simulink model "PID_controller_lat_stage1_plot"  (R2019a)
settings: Solver=VariableStepAuto  StartTime=0.0  StopTime=100  FixedStep=1e-4  RelTol=1e-5
undefined symbols (not defined in the file): sys
libraries: aerolibactuator x1, simulink x1
settings Model: Creator=tyson  LastModifiedBy=tyson
settings DebuggingCC: TimeAdjustmentMsg=warning

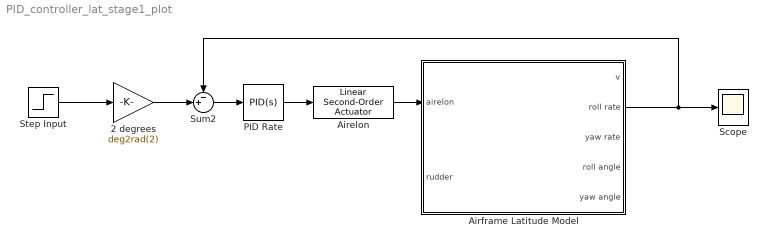
== system PID_controller_lat_stage1_plot ==
  2 degrees : Gain  Gain=deg2rad(2)
  Airelon : aerolibactuator/Linear Second-Order Actuator  wn_fin=actuators.naturalFreq  z_fin=actuators.dampingRatio  fin_act_0=0  fin_act_vel=0
      settings: SourceProductName=Aerospace Blockset  SourceProductBaseCode=AE
  Airframe Latitude Model : Subsystem
      mask Display: image('/home/tyson/Dropbox/Academic/4th Year/ELEN4011/matlab/icons/airframe_lat.png');
  PID Rate : simulink/Continuous/PID Controller  Controller=PID  Form=Parallel  TimeDomain=Continuous-time  SampleTime=-1  IntegratorMethod=Forward Euler  FilterMethod=Forward Euler  ControllerParametersSource=internal  P=0.088381890868231  I=0.0632480324268729  D=-0.40850773748129  UseFilter=on  N=0.167390609816389  TunerSelectOption=Transfer Function Based (PID Tuner App)  InitialConditionSource=internal  InitialConditionForIntegrator=0  InitialConditionForFilter=0  DifferentiatorICPrevScaledInput=0  ExternalReset=none  TrackingMode=off  Kt=1  LimitOutput=off  UpperSaturationLimit=pi  LowerSaturationLimit=-pi  LinearizeAsGain=on  AntiWindupMode=clamping  Kb=1  POutMin=[]  POutMax=[]  IOutMin=[]  IOutMax=[]  DOutMin=[]  DOutMax=[]  NOutMin=[]  NOutMax=[]  SumOutMin=[]  SumOutMax=[]  SaturationOutMin=[]  SaturationOutMax=[]  PParamMin=[]  PParamMax=[]  IParamMin=[]  IParamMax=[]  DParamMin=[]  DParamMax=[]  NParamMin=[]  NParamMax=[]  KbParamMin=[]  KbParamMax=[]  KtParamMin=[]  KtParamMax=[]  KbOutMin=[]  KbOutMax=[]  KtOutMin=[]  KtOutMax=[]  IntegratorOutMin=[]  IntegratorOutMax=[]  FilterOutMin=[]  FilterOutMax=[]  SumI1OutMin=[]  SumI1OutMax=[]  SumI2OutMin=[]  SumI2OutMax=[]  SumI3OutMin=[]  SumI3OutMax=[]  SumI4OutMin=[]  SumI4OutMax=[]  SumDOutMin=[]  SumDOutMax=[]  DifferentiatorOutMin=[]  DifferentiatorOutMax=[]  FilterDiffOutCoefMin=[]  FilterDiffOutCoefMax=[]  ReciprocalOutMin=[]  ReciprocalOutMax=[]  SumDenOutMin=[]  SumDenOutMax=[]  SumNumOutMin=[]  SumNumOutMax=[]  DivideOutMin=[]  DivideOutMax=[]  IntegratorContinuousStateAttributes=''  IntegratorStateMustResolveToSignalObject=off  IntegratorRTWStateStorageClass=Auto  FilterContinuousStateAttributes=''  FilterStateMustResolveToSignalObject=off  FilterRTWStateStorageClass=Auto  ParallelPVariant=InternalParameters  IdealPVariant=Disabled  IVariant=InternalParameters  DVariant=InternalParameters  IntegratorVariant=Continuous  SatVariant=Disabled  AWVariant=Passthrough  PCopyVariant=Disabled  TRVariant=Disabled  FdbkBlocksVariant=Forward  IdealPFdbkVariant=Disabled  SatFdbkVariant=Disabled  DerivativeFilterVariant=ContFilter  NVariant=InternalParameters  NCopyVariant=Disabled  FilterICVariant=InternalICsFilter  IntegratorICVariant=InternalICs  ExternalResetVariant=Disabled  TRSumVariant=Passthrough  SumFdbkVariant=Disabled  SumVariant=Sum_PID
  Scope : Scope
  Step Input : Step
  Sum2 : Sum  Inputs=-+|
  wires:
  Step Input/1 -> 2 degrees/1
  Airelon/1 -> Airframe Latitude Model/1(airelon)
  Sum2/1 -> PID Rate/1
  2 degrees/1 -> Sum2/2
  Airframe Latitude Model/2(roll rate) -> Scope/1, Sum2/1
  PID Rate/1 -> Airelon/1

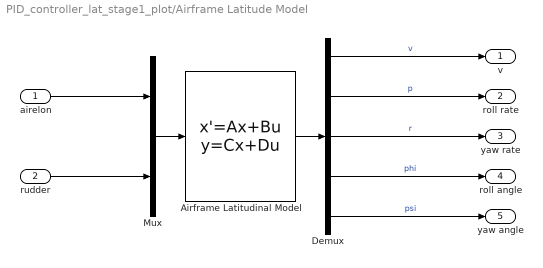
== system PID_controller_lat_stage1_plot/Airframe Latitude Model ==
  airelon : Inport
  rudder : Inport  Port=2
  Airframe Latitudinal Model : StateSpace  A=sys.lat.A  B=sys.lat.B  C=sys.lat.C  D=sys.lat.D  InitialCondition=0
  Demux : Demux  Outputs=5
  Mux : Mux  Inputs=2
  v : Outport
  roll rate : Outport  Port=2
  yaw rate : Outport  Port=3
  roll angle : Outport  Port=4
  yaw angle : Outport  Port=5
  wires:
  rudder/1 -> Mux/2
  Demux/4 -> roll angle/1  "phi"
  Demux/3 -> yaw rate/1  "r"
  Mux/1 -> Airframe Latitudinal Model/1
  Airframe Latitudinal Model/1 -> Demux/1
  Demux/1 -> v/1  "v"
  Demux/2 -> roll rate/1  "p"
  Demux/5 -> yaw angle/1  "psi"
  airelon/1 -> Mux/1
